simulink model "working_kalman"  (R2025b)
settings: Solver=FixedStepDiscrete  StartTime=0.0  StopTime=+inf  FixedStep=simulink_Ts  RelTol=1e-3  EnableMultiTasking=on
InitFcn:
  | InitSensorFusion
values from neighbouring files (symbols this model uses):
  acc_calib_matrix = [0.9990,0.0039,0.0028;4.2507e-04,0.9990,-0.0085;0.0015,0.0090,0.9997]    [InitSensorFusion.m]
  avg_order = 2    [InitSensorFusion.m]
  calibration_time = 10    [InitSensorFusion.m]
  d = 0.15*sqrt(2)/2    [InitSensorFusion.m]
  friction_offset = 0.0001    [InitSensorFusion.m]
  friction_slope = 20e-6    (= 2e-05)    [InitSensorFusion.m]
  g = 9.81    [InitSensorFusion.m]
  ground_true_g = 9.81275    [InitSensorFusion.m]
  Ic0 = Is0 + Iw0 - Iwg    [InitSensorFusion.m]
  ICM42_gyr_offset = [-0.1319, -0.6878, 0.1737]    [InitSensorFusion.m]
  ICM42_params = SUPER_PARAMS    [InitSensorFusion.m]
  init_acc_bias = [-0.0076;0.0233;0.0477]    [InitSensorFusion.m]
  init_P = P_initial    [InitSensorFusion.m]
  init_rot_quat = [0 0 0 1]'    [InitSensorFusion.m]
  Iwg = 315e-6    (= 0.000315)    [InitSensorFusion.m]
  kalman_Ts = 0.01    [InitSensorFusion.m]
  KV = 330    [InitSensorFusion.m]
  mc = mw + ms    (= 0.75)    [InitSensorFusion.m]
  sensor_Ts = 0.01    [InitSensorFusion.m]
  simulink_Ts = 0.01    [InitSensorFusion.m]
  stateInit = StateEnum.Initialization    [InitSensorFusion.m]
undefined symbols (not defined in the file or in its folder): acc_init_bias, init_time, StateEnum
libraries: mbedblockslib x25, simulink x12, nucleoutilitieslib x10, stmnucleof7lib x7, canmsglib x6, simulink_extras x2, visionstatistics x2
(part 2 of 2)

== system working_kalman/Sensor Calibration and Averaging/Subsystem2 ==
  g_vector : Inport
  Enable : EnablePort
  2-D Mean3 : visionstatistics/2-D Mean  run=on  reset_popup=Rising edge  directionMode=Each row  dimension=1  treatSBRowAsCol=on  outputLastDataTypeStr=Inherit: Same as accumulator  accumMode=Binary point scaling  accumWordLength=32  accumFracLength=0  accumLastDataTypeStr=fixdt([],32,0)  roiEnable=off  roiType=Rectangles  roiPortion=Entire ROI  roiOutput=Individual statistics for each ROI  roiFlag=off  roundingMode=Floor  overflowMode=off  accumDataTypeStr=fixdt([],32,0)  outputDataTypeStr=Inherit: Same as accumulator  outputMin=[]  outputMax=[]
  Cast To Boolean : DataTypeConversion  OutDataTypeStr=boolean  SaturateOnIntegerOverflow=off  RndMeth=Floor
  MATLAB Function1 : MATLAB Function  TreatAsAtomicUnit=on
  Sum : Sum  Inputs=|-+
  Sum of Elements : Sum  Inputs=+
  ground_true_g_vector : Constant  Value=[0; 0; -ground_true_g]  SampleTime=simulink_Ts
  g_mean : Outport
  acc_bias : Outport  Port=2
  wires:
  2-D Mean3/1 -> g_mean/1
  g_vector/1 -> MATLAB Function1/1(g_vector), Sum of Elements/1, Sum/2
  MATLAB Function1/1(g_scalar) -> 2-D Mean3/1
  Sum of Elements/1 -> Cast To Boolean/1
  Cast To Boolean/1 -> 2-D Mean3/2
  ground_true_g_vector/1 -> Sum/1
  Sum/1 -> acc_bias/1

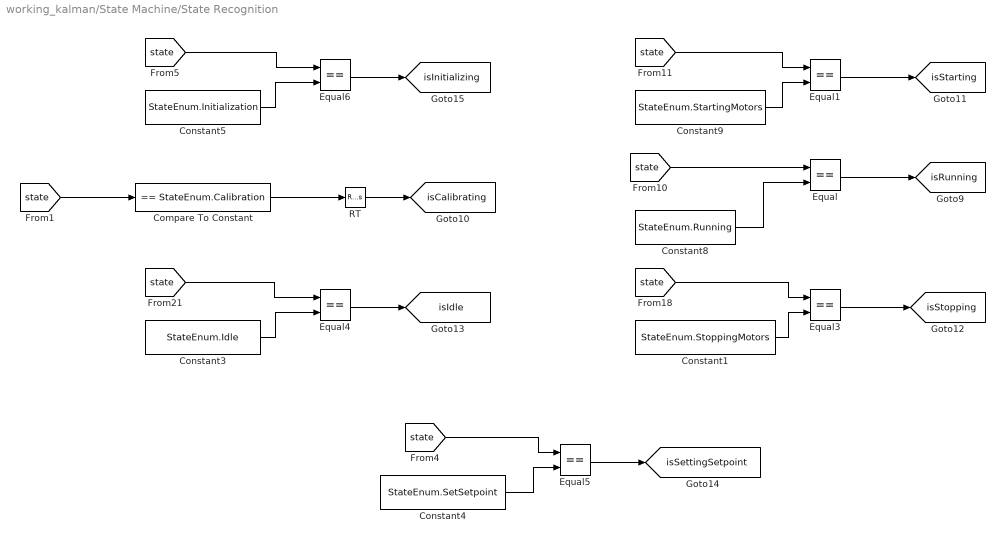
== system working_kalman/State Machine/State Recognition ==
  Compare To Constant : simulink/Logic and Bit Operations/Compare To Constant  relop===  const=StateEnum.Calibration  OutDataTypeStr=boolean
  Constant1 : Constant  Value=StateEnum.StoppingMotors  SampleTime=simulink_Ts
  Constant3 : Constant  Value=StateEnum.Idle  SampleTime=simulink_Ts
  Constant4 : Constant  Value=StateEnum.SetSetpoint  SampleTime=simulink_Ts
  Constant5 : Constant  Value=StateEnum.Initialization  SampleTime=simulink_Ts
  Constant8 : Constant  Value=StateEnum.Running  SampleTime=simulink_Ts
  Constant9 : Constant  Value=StateEnum.StartingMotors  SampleTime=simulink_Ts
  Equal{,1,3..6} (6 alike) : RelationalOperator  Operator===  OutDataTypeStr=boolean  RndMeth=Simplest  InputSameDT=off
  RT : RateTransition  OutPortSampleTime=sensor_Ts
  tag scope: isCalibrating=global, isIdle=global, isInitializing=global, isRunning=global, isSettingSetpoint=global, isStarting=global, isStopping=global
  wires:
  [state] -> Equal4/1
  Equal6/1 -> [isInitializing]
  [state] -> Equal1/1
  Constant9/1 -> Equal1/2
  Constant4/1 -> Equal5/2
  Constant8/1 -> Equal/2
  [state] -> Equal/1
  Equal4/1 -> [isIdle]
  Constant3/1 -> Equal4/2
  Constant5/1 -> Equal6/2
  Equal1/1 -> [isStarting]
  Equal/1 -> [isRunning]
  Constant1/1 -> Equal3/2
  [state] -> Equal3/1
  Equal5/1 -> [isSettingSetpoint]
  Equal3/1 -> [isStopping]
  [state] -> Equal6/1
  [state] -> Equal5/1
  [state] -> Compare To Constant/1
  Compare To Constant/1 -> RT/1
  RT/1 -> [isCalibrating]

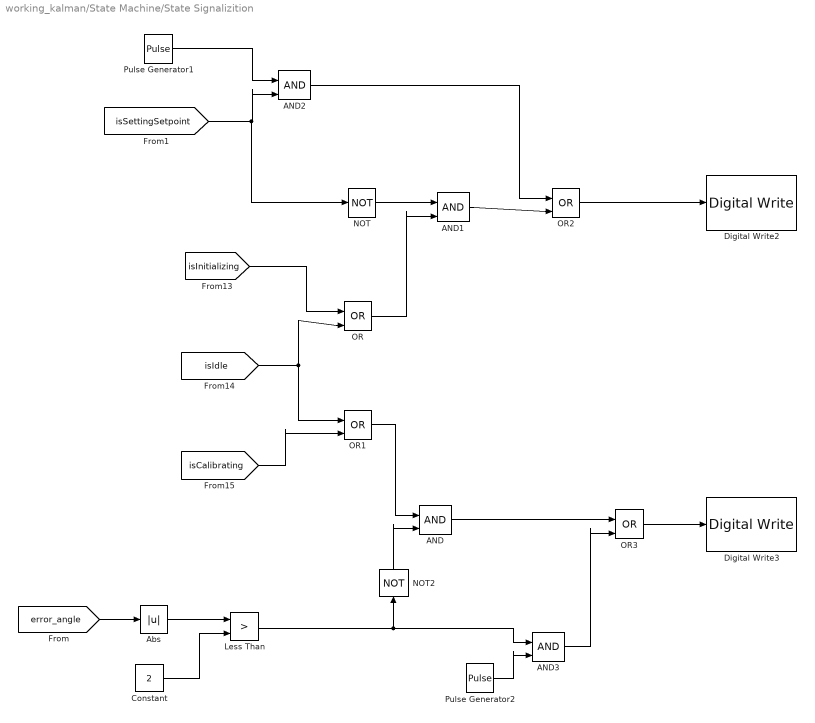
== system working_kalman/State Machine/State Signalizition ==
  AND{,1..3} (4 alike) : Logic  IconShape=distinctive  AllPortsSameDT=off  OutDataTypeStr=boolean
  Abs : Abs  SaturateOnIntegerOverflow=off
  Constant : Constant  Value=2
  Digital Write2 : mbedblockslib/Digital Write  Pin=LED3  Direction=output
      settings: LibrarySourceBlock=stmnucleorootlib/Common/Digital Write
  Digital Write3 : mbedblockslib/Digital Write  Pin=LED2  Direction=output
      settings: LibrarySourceBlock=stmnucleorootlib/Common/Digital Write
  Less Than : RelationalOperator  Operator=>  OutDataTypeStr=boolean  RndMeth=Simplest  InputSameDT=off
  NOT : Logic  Operator=NOT  IconShape=distinctive  AllPortsSameDT=off  OutDataTypeStr=boolean
  NOT2 : Logic  Operator=NOT  IconShape=distinctive  AllPortsSameDT=off  OutDataTypeStr=boolean
  OR{,1..3} (4 alike) : Logic  Operator=OR  IconShape=distinctive  AllPortsSameDT=off  OutDataTypeStr=boolean
  Pulse Generator1 : DiscretePulseGenerator  PulseType=Time based  Period=0.1  PulseWidth=50
  Pulse Generator2 : DiscretePulseGenerator  PulseType=Time based  Period=0.1  PulseWidth=50
  wires:
  [isInitializing] -> OR/1
  [isCalibrating] -> OR1/2
  [isIdle] -> OR1/1, OR/2
  OR1/1 -> AND/1
  OR/1 -> AND1/2
  Abs/1 -> Less Than/1
  Constant/1 -> Less Than/2
  Pulse Generator1/1 -> AND2/1
  [isSettingSetpoint] -> NOT/1, AND2/2
  NOT/1 -> AND1/1
  AND1/1 -> OR2/2
  AND2/1 -> OR2/1
  OR2/1 -> Digital Write2/1
  [error_angle] -> Abs/1
  Less Than/1 -> AND3/1, NOT2/1
  Pulse Generator2/1 -> AND3/2
  AND/1 -> OR3/1
  AND3/1 -> OR3/2
  OR3/1 -> Digital Write3/1
  NOT2/1 -> AND/2

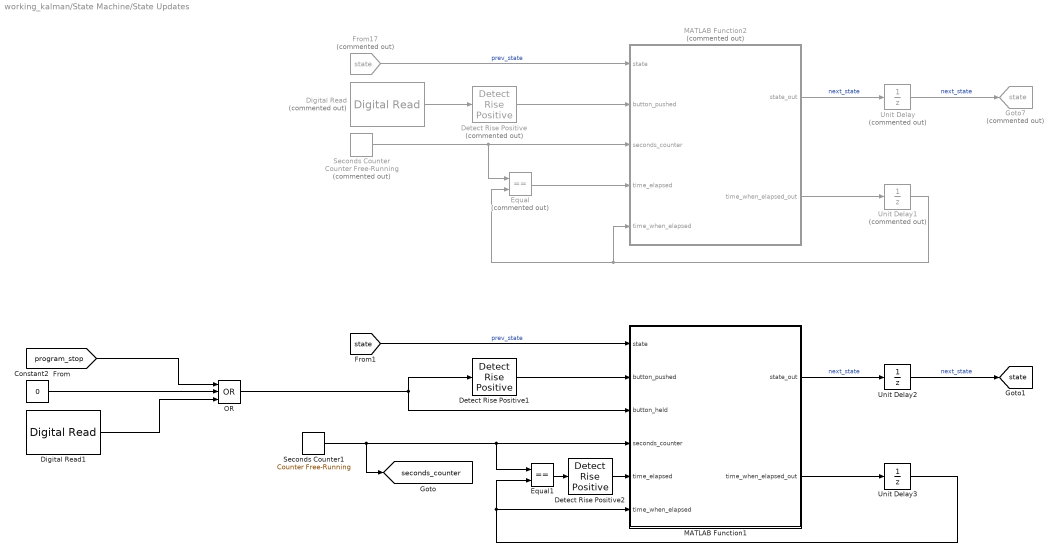
== system working_kalman/State Machine/State Updates ==
  Constant2 : Constant  Value=0
  Detect Rise Positive : simulink/Logic and Bit Operations/Detect Rise Positive  Commented=on  vinit=0  OutDataTypeStr=boolean
  Detect Rise Positive1 : simulink/Logic and Bit Operations/Detect Rise Positive  vinit=0  OutDataTypeStr=boolean
  Detect Rise Positive2 : simulink/Logic and Bit Operations/Detect Rise Positive  vinit=0  OutDataTypeStr=boolean
  Digital Read : mbedblockslib/Digital Read  Commented=on  Pin=D0  Direction=input  SampleTime=0.1
      settings: LibrarySourceBlock=stmnucleorootlib/Common/Digital Read
  Digital Read1 : mbedblockslib/Digital Read  Pin=PC_13  Direction=input  SampleTime=simulink_Ts
      settings: LibrarySourceBlock=stmnucleorootlib/Common/Digital Read
  Equal : RelationalOperator  Commented=on  Operator===  OutDataTypeStr=boolean  RndMeth=Simplest  InputSameDT=off
  Equal1 : RelationalOperator  Operator===  OutDataTypeStr=boolean  RndMeth=Simplest  InputSameDT=off
  From17 : From  Commented=on  GotoTag=state  TagVisibility=global
  Goto7 : Goto  Commented=on  GotoTag=state  TagVisibility=global
  MATLAB Function1 : MATLAB Function  TreatAsAtomicUnit=on  SystemSampleTime=simulink_Ts
  MATLAB Function2 : MATLAB Function  Commented=on  TreatAsAtomicUnit=on
  OR : Logic  Operator=OR  Inputs=3  IconShape=distinctive  AllPortsSameDT=off  OutDataTypeStr=boolean
  Seconds Counter : simulink/Sources/Counter Free-Running  Commented=on  NumBits=16  tsamp=1
  Seconds Counter1 : simulink/Sources/Counter Free-Running  NumBits=16  tsamp=1
  Unit Delay : UnitDelay  Commented=on  InitialCondition=stateInit  SampleTime=-1  HasFrameUpgradeWarning=on
  Unit Delay1 : UnitDelay  Commented=on  InitialCondition=init_time  SampleTime=-1  HasFrameUpgradeWarning=on
  Unit Delay2 : UnitDelay  InitialCondition=stateInit  SampleTime=simulink_Ts  HasFrameUpgradeWarning=on
  Unit Delay3 : UnitDelay  InitialCondition=init_time  SampleTime=simulink_Ts  HasFrameUpgradeWarning=on
  tag scope: seconds_counter=global, state=global
  wires:
  Unit Delay/1 -> Goto7/1  "next_state"
  Digital Read/1 -> Detect Rise Positive/1
  From17/1 -> MATLAB Function2/1(state)  "prev_state"
  Detect Rise Positive/1 -> MATLAB Function2/2(button_pushed)
  Seconds Counter/1 -> Equal/1, MATLAB Function2/3(seconds_counter)
  Equal/1 -> MATLAB Function2/4(time_elapsed)
  MATLAB Function2/2(time_when_elapsed_out) -> Unit Delay1/1
  Unit Delay1/1 -> MATLAB Function2/5(time_when_elapsed), Equal/2
  MATLAB Function2/1(state_out) -> Unit Delay/1  "next_state"
  Equal1/1 -> Detect Rise Positive2/1
  Detect Rise Positive1/1 -> MATLAB Function1/2(button_pushed)
  [state] -> MATLAB Function1/1(state)  "prev_state"
  Unit Delay2/1 -> [state]  "next_state"
  MATLAB Function1/1(state_out) -> Unit Delay2/1  "next_state"
  Seconds Counter1/1 -> Equal1/1, MATLAB Function1/4(seconds_counter), [seconds_counter]
  MATLAB Function1/2(time_when_elapsed_out) -> Unit Delay3/1
  Unit Delay3/1 -> Equal1/2, MATLAB Function1/6(time_when_elapsed)
  Constant2/1 -> OR/2
  [program_stop] -> OR/1
  Digital Read1/1 -> OR/3
  OR/1 -> Detect Rise Positive1/1, MATLAB Function1/3(button_held)
  Detect Rise Positive2/1 -> MATLAB Function1/5(time_elapsed)

== system working_kalman/CAN communication with B-G431-ESC1/Receive CAN Messages/Subsystem1 ==
  In1 : Inport
  Enable : EnablePort
  Byte Unpack : nucleoutilitieslib/Byte Unpack  dimensions={[2]}  datatypes={'single'}  byteAlign=1  blockPlatform=nucleo
  Out1 : Outport
  wires:
  Byte Unpack/1 -> Out1/1
  In1/1 -> Byte Unpack/1

== system working_kalman/CAN communication with B-G431-ESC1/Receive CAN Messages/Subsystem2 ==
  In1 : Inport
  Enable : EnablePort
  Byte Unpack : nucleoutilitieslib/Byte Unpack  dimensions={[2]}  datatypes={'single'}  byteAlign=1  blockPlatform=nucleo
  Out1 : Outport
  wires:
  Byte Unpack/1 -> Out1/1
  In1/1 -> Byte Unpack/1

== system working_kalman/CAN communication with B-G431-ESC1/Send CAN Messages/CAN_send ==
  data : Inport
  ID : Inport  Port=2
  Trigger : TriggerPort  VariantControl=(inherit)  PortDimensions=1
  CAN Pack : canmsglib/CAN Pack  MsgList=(none)  MsgName=LED_set  MsgIDType=Standard (11-bit identifier)  MsgIdentifier=hex2dec('7F3')  CANIDInput=on  MsgLength=8  Remote=off  ApplyMinMax=off  BusOutput=on  SignalInfo={}
      settings: LibrarySourceBlock=nucleoutilitieslib/CAN Pack  DataFormat=raw data
  CAN Transmit : stmnucleof7lib/CAN Transmit  CANModule=1  IdentifierType=Standard (11-bit identifier)  MsgId=hex2dec('7F3')  MsgLen=8  OutputStatus=on  RemoteFrame=off
      settings: DataFormat=CAN Message
  wires:
  CAN Pack/1 -> CAN Transmit/1
  data/1 -> CAN Pack/1
  ID/1 -> CAN Pack/2

== system working_kalman/CAN communication with B-G431-ESC1/Send CAN Messages/CAN_send1 ==
  data : Inport
  ID : Inport  Port=2
  Trigger : TriggerPort  VariantControl=(inherit)  PortDimensions=1
  CAN Pack : canmsglib/CAN Pack  MsgList=(none)  MsgName=LED_set  MsgIDType=Standard (11-bit identifier)  MsgIdentifier=hex2dec('7F3')  CANIDInput=on  MsgLength=8  Remote=off  ApplyMinMax=off  BusOutput=on  SignalInfo={}
      settings: LibrarySourceBlock=nucleoutilitieslib/CAN Pack  DataFormat=raw data
  CAN Transmit : stmnucleof7lib/CAN Transmit  CANModule=1  IdentifierType=Standard (11-bit identifier)  MsgId=hex2dec('7F3')  MsgLen=8  OutputStatus=on  RemoteFrame=off
      settings: DataFormat=CAN Message
  wires:
  CAN Pack/1 -> CAN Transmit/1
  data/1 -> CAN Pack/1
  ID/1 -> CAN Pack/2

== system working_kalman/CAN communication with B-G431-ESC1/Send CAN Messages/CAN_send2 ==
  data : Inport
  ID : Inport  Port=2
  Trigger : TriggerPort  VariantControl=(inherit)  PortDimensions=1
  CAN Pack : canmsglib/CAN Pack  MsgList=(none)  MsgName=LED_set  MsgIDType=Standard (11-bit identifier)  MsgIdentifier=hex2dec('7F3')  CANIDInput=on  MsgLength=8  Remote=off  ApplyMinMax=off  BusOutput=on  SignalInfo={}
      settings: LibrarySourceBlock=nucleoutilitieslib/CAN Pack  DataFormat=raw data
  CAN Transmit : stmnucleof7lib/CAN Transmit  CANModule=1  IdentifierType=Standard (11-bit identifier)  MsgId=hex2dec('7F3')  MsgLen=8  OutputStatus=on  RemoteFrame=off
      settings: DataFormat=CAN Message
  wires:
  CAN Pack/1 -> CAN Transmit/1
  data/1 -> CAN Pack/1
  ID/1 -> CAN Pack/2

== system working_kalman/CAN communication with B-G431-ESC1/Send CAN Messages/CAN_send3 ==
  data : Inport
  ID : Inport  Port=2
  Trigger : TriggerPort  VariantControl=(inherit)  PortDimensions=1
  CAN Pack : canmsglib/CAN Pack  MsgList=(none)  MsgName=LED_set  MsgIDType=Standard (11-bit identifier)  MsgIdentifier=hex2dec('7F3')  CANIDInput=on  MsgLength=8  Remote=off  ApplyMinMax=off  BusOutput=on  SignalInfo={}
      settings: LibrarySourceBlock=nucleoutilitieslib/CAN Pack  DataFormat=raw data
  CAN Transmit : stmnucleof7lib/CAN Transmit  CANModule=1  IdentifierType=Standard (11-bit identifier)  MsgId=hex2dec('7F3')  MsgLen=8  OutputStatus=on  RemoteFrame=off
      settings: DataFormat=CAN Message
  wires:
  CAN Pack/1 -> CAN Transmit/1
  data/1 -> CAN Pack/1
  ID/1 -> CAN Pack/2

== system working_kalman/CAN communication with B-G431-ESC1/Send CAN Messages/CAN_send4 ==
  data : Inport
  ID : Inport  Port=2
  Trigger : TriggerPort  VariantControl=(inherit)  PortDimensions=1
  CAN Pack : canmsglib/CAN Pack  MsgList=(none)  MsgName=LED_set  MsgIDType=Standard (11-bit identifier)  MsgIdentifier=hex2dec('7F3')  CANIDInput=on  MsgLength=8  Remote=off  ApplyMinMax=off  BusOutput=on  SignalInfo={}
      settings: LibrarySourceBlock=nucleoutilitieslib/CAN Pack  DataFormat=raw data
  CAN Transmit : stmnucleof7lib/CAN Transmit  CANModule=1  IdentifierType=Standard (11-bit identifier)  MsgId=hex2dec('7F3')  MsgLen=8  OutputStatus=on  RemoteFrame=off
      settings: DataFormat=CAN Message
  wires:
  CAN Pack/1 -> CAN Transmit/1
  data/1 -> CAN Pack/1
  ID/1 -> CAN Pack/2

== system working_kalman/CAN communication with B-G431-ESC1/Send CAN Messages/CAN_send5 ==
  data : Inport
  ID : Inport  Port=2
  Trigger : TriggerPort  VariantControl=(inherit)  PortDimensions=1
  CAN Pack : canmsglib/CAN Pack  MsgList=(none)  MsgName=LED_set  MsgIDType=Standard (11-bit identifier)  MsgIdentifier=hex2dec('7F3')  CANIDInput=on  MsgLength=8  Remote=off  ApplyMinMax=off  BusOutput=on  SignalInfo={}
      settings: LibrarySourceBlock=nucleoutilitieslib/CAN Pack  DataFormat=raw data
  CAN Transmit : stmnucleof7lib/CAN Transmit  CANModule=1  IdentifierType=Standard (11-bit identifier)  MsgId=hex2dec('7F3')  MsgLen=8  OutputStatus=on  RemoteFrame=off
      settings: DataFormat=CAN Message
  wires:
  CAN Pack/1 -> CAN Transmit/1
  data/1 -> CAN Pack/1
  ID/1 -> CAN Pack/2

== system working_kalman/CAN communication with B-G431-ESC1/Send CAN Messages/Set_LED ==
  Cast To Double : DataTypeConversion  OutDataTypeStr=uint8  SaturateOnIntegerOverflow=off  RndMeth=Floor
  Constant : Constant  Value=zeros(1,7)
  Constant5 : Constant  Value=hex2dec('7F3')
  Pulse Generator1 : DiscretePulseGenerator  PulseType=Time based  Period=1  PulseWidth=50
  Vector Concatenate : Concatenate
  data : Outport
  ID : Outport  Port=2
  wires:
  Constant5/1 -> ID/1
  Pulse Generator1/1 -> Vector Concatenate/1
  Vector Concatenate/1 -> Cast To Double/1
  Constant/1 -> Vector Concatenate/2
  Cast To Double/1 -> data/1

== system working_kalman/CAN communication with B-G431-ESC1/Send CAN Messages/Set_speed ==
  Byte Pack1 : nucleoutilitieslib/Byte Pack  datatypes={'uint16'}  byteAlign=1  blockPlatform=nucleo
  Byte Pack2 : nucleoutilitieslib/Byte Pack  datatypes={'single'}  byteAlign=1  blockPlatform=nucleo
  Constant1 : Constant  Value=[0,0]  OutDataTypeStr=uint8  SampleTime=-1
  Constant5 : Constant  Value=hex2dec('023')
  Vector Concatenate3 : Concatenate  NumInputs=3
  time_ramp [ms] : Constant  Value=0  OutDataTypeStr=uint16
  data : Outport
  ID : Outport  Port=2
  wires:
  Vector Concatenate3/1 -> data/1
  Constant5/1 -> ID/1
  Byte Pack2/1 -> Vector Concatenate3/1
  Byte Pack1/1 -> Vector Concatenate3/2
  Constant1/1 -> Vector Concatenate3/3
  time_ramp [ms]/1 -> Byte Pack1/1
  [ramp_speed] -> Byte Pack2/1

== system working_kalman/CAN communication with B-G431-ESC1/Send CAN Messages/Set_speed1 ==
  In1 : Inport
  Byte Pack1 : nucleoutilitieslib/Byte Pack  datatypes={'uint16'}  byteAlign=1  blockPlatform=nucleo
  Byte Pack2 : nucleoutilitieslib/Byte Pack  datatypes={'single'}  byteAlign=1  blockPlatform=nucleo
  Constant1 : Constant  Value=[0,0]  OutDataTypeStr=uint8  SampleTime=-1
  Constant5 : Constant  Value=hex2dec('023')
  Sum : Sum  Inputs=++|
  Vector Concatenate3 : Concatenate  NumInputs=3
  final_speed [rpm] : Constant  Value=1200  OutDataTypeStr=single
  time_ramp [ms] : Constant  Value=500  OutDataTypeStr=uint16
  data : Outport
  ID : Outport  Port=2
  wires:
  time_ramp [ms]/1 -> Byte Pack1/1
  Constant1/1 -> Vector Concatenate3/3
  Byte Pack1/1 -> Vector Concatenate3/2
  Byte Pack2/1 -> Vector Concatenate3/1
  Constant5/1 -> ID/1
  Vector Concatenate3/1 -> data/1
  final_speed [rpm]/1 -> Sum/2
  Sum/1 -> Byte Pack2/1
  In1/1 -> Sum/1  "angle_dep_spd"

== system working_kalman/CAN communication with B-G431-ESC1/Send CAN Messages/Set_torque ==
  Byte Pack1 : nucleoutilitieslib/Byte Pack  datatypes={'uint16'}  byteAlign=1  blockPlatform=nucleo
  Byte Pack2 : nucleoutilitieslib/Byte Pack  datatypes={'single'}  byteAlign=1  blockPlatform=nucleo
  Cast : DataTypeConversion  OutDataTypeStr=single  SaturateOnIntegerOverflow=off  RndMeth=Floor
  Constant1 : Constant  Value=[0,0]  OutDataTypeStr=uint8  SampleTime=-1
  Constant5 : Constant  Value=hex2dec('043')
  Vector Concatenate3 : Concatenate  NumInputs=3
  time_ramp [ms] : Constant  Value=0  OutDataTypeStr=uint16  SampleTime=-1
  data : Outport
  ID : Outport  Port=2
  wires:
  time_ramp [ms]/1 -> Byte Pack1/1
  Constant1/1 -> Vector Concatenate3/3
  Byte Pack1/1 -> Vector Concatenate3/2
  Byte Pack2/1 -> Vector Concatenate3/1
  Constant5/1 -> ID/1
  Vector Concatenate3/1 -> data/1
  [ramp_torque] -> Cast/1  "reference_torque [A]"
  Cast/1 -> Byte Pack2/1

== system working_kalman/CAN communication with B-G431-ESC1/Send CAN Messages/Start_Motor ==
  Constant3 : Constant  Value=[1,0,0,0,0,0,0,0]  OutDataTypeStr=uint8  SampleTime=-1
  Constant4 : Constant  Value=hex2dec('033')
  data : Outport
  ID : Outport  Port=2
  wires:
  Constant3/1 -> data/1
  Constant4/1 -> ID/1

== system working_kalman/CAN communication with B-G431-ESC1/Send CAN Messages/Stop_Motor ==
  Byte Pack1 : nucleoutilitieslib/Byte Pack  datatypes={'uint16'}  byteAlign=1  blockPlatform=nucleo
  Byte Pack2 : nucleoutilitieslib/Byte Pack  datatypes={'single'}  byteAlign=1  blockPlatform=nucleo
  Constant1 : Constant  Value=[0,0]  OutDataTypeStr=uint8  SampleTime=-1
  Constant3 : Constant  Value=[0,0,0,0,0,0,0,0]  OutDataTypeStr=uint8  SampleTime=-1
  Constant4 : Constant  Value=hex2dec('033')
  Constant5 : Constant  Value=hex2dec('023')
  Vector Concatenate3 : Concatenate  NumInputs=3
  final_speed [rpm] : Constant  Value=-1200  OutDataTypeStr=single
  time_ramp [ms] : Constant  OutDataTypeStr=uint16
  data : Outport
  ID : Outport  Port=2
  wires:
  Byte Pack2/1 -> Vector Concatenate3/1
  final_speed [rpm]/1 -> Byte Pack2/1
  time_ramp [ms]/1 -> Byte Pack1/1
  Byte Pack1/1 -> Vector Concatenate3/2
  Constant1/1 -> Vector Concatenate3/3
  Constant4/1 -> ID/1
  Constant3/1 -> data/1

== system working_kalman/ICM20948/Read sensing data/Subsystem ==
  In1 : Inport
  Add Constant : Bias  Bias=36.53  SaturateOnIntegerOverflow=off
  Cast To Double : DataTypeConversion  OutDataTypeStr=double  SaturateOnIntegerOverflow=off  RndMeth=Floor
  Gain7 : Gain  Gain=1/340
  Out1 : Outport
  wires:
  Gain7/1 -> Add Constant/1  "Temp"
  Add Constant/1 -> Out1/1
  In1/1 -> Cast To Double/1
  Cast To Double/1 -> Gain7/1

== system working_kalman/ICM20948/Read sensing data/Subsystem1 ==
  In1 : Inport
  8g range : Gain  Gain=9.81275/4096
  Cast To Double : DataTypeConversion  OutDataTypeStr=double  SaturateOnIntegerOverflow=off  RndMeth=Floor
  Offset : Bias  SaturateOnIntegerOverflow=off
  Out1 : Outport
  wires:
  Cast To Double/1 -> 8g range/1
  Offset/1 -> Out1/1
  In1/1 -> Cast To Double/1
  8g range/1 -> Offset/1  "Acc_Z"

== system working_kalman/ICM20948/Read sensing data/Subsystem2 ==
  In1 : Inport
  8g range : Gain  Gain=9.81275/4096
  Cast To Double : DataTypeConversion  OutDataTypeStr=double  SaturateOnIntegerOverflow=off  RndMeth=Floor
  Offset : Bias  SaturateOnIntegerOverflow=off
  Out1 : Outport
  wires:
  8g range/1 -> Offset/1  "Acc_Z"
  In1/1 -> Cast To Double/1
  Offset/1 -> Out1/1
  Cast To Double/1 -> 8g range/1

== system working_kalman/ICM20948/Read sensing data/Subsystem3 ==
  In1 : Inport
  8g range : Gain  Gain=9.81275/4096
  Cast To Double : DataTypeConversion  OutDataTypeStr=double  SaturateOnIntegerOverflow=off  RndMeth=Floor
  Offset : Bias  SaturateOnIntegerOverflow=off
  Out1 : Outport
  wires:
  8g range/1 -> Offset/1  "Acc_Z"
  In1/1 -> Cast To Double/1
  Offset/1 -> Out1/1
  Cast To Double/1 -> 8g range/1

== system working_kalman/ICM20948/Read sensing data/Subsystem4 ==
  In1 : Inport
  +-500 °/s range : Gain  Gain=1/65.5
  Cast To Double : DataTypeConversion  OutDataTypeStr=double  SaturateOnIntegerOverflow=off  RndMeth=Floor
  Offset : Bias  SaturateOnIntegerOverflow=off
  Out1 : Outport
  wires:
  Offset/1 -> Out1/1
  +-500 °/s range/1 -> Offset/1  "Acc_Z"
  Cast To Double/1 -> +-500 °/s range/1
  In1/1 -> Cast To Double/1

== system working_kalman/ICM20948/Read sensing data/Subsystem5 ==
  In1 : Inport
  +-500 °/s range : Gain  Gain=1/65.5
  Cast To Double : DataTypeConversion  OutDataTypeStr=double  SaturateOnIntegerOverflow=off  RndMeth=Floor
  Offset : Bias  SaturateOnIntegerOverflow=off
  Out1 : Outport
  wires:
  Offset/1 -> Out1/1
  +-500 °/s range/1 -> Offset/1  "Acc_Z"
  Cast To Double/1 -> +-500 °/s range/1
  In1/1 -> Cast To Double/1

== system working_kalman/ICM20948/Read sensing data/Subsystem6 ==
  In1 : Inport
  +-500 °/s range : Gain  Gain=1/65.5
  Cast To Double : DataTypeConversion  OutDataTypeStr=double  SaturateOnIntegerOverflow=off  RndMeth=Floor
  Offset : Bias  SaturateOnIntegerOverflow=off
  Out1 : Outport
  wires:
  Offset/1 -> Out1/1
  +-500 °/s range/1 -> Offset/1  "Acc_Z"
  Cast To Double/1 -> +-500 °/s range/1
  In1/1 -> Cast To Double/1

== system working_kalman/ICM42688-P/Measurement/Subsystem ==
  In1 : Inport
  Add Constant : Bias  Bias=25  SaturateOnIntegerOverflow=off
  Cast To Double : DataTypeConversion  OutDataTypeStr=double  SaturateOnIntegerOverflow=off  RndMeth=Floor
  Gain7 : Gain  Gain=1/132.48
  Out1 : Outport
  wires:
  Gain7/1 -> Add Constant/1  "Temp"
  Add Constant/1 -> Out1/1
  In1/1 -> Cast To Double/1
  Cast To Double/1 -> Gain7/1

== system working_kalman/ICM42688-P/Measurement/Subsystem1 ==
  In1 : Inport
  8g range : Gain  Gain=9.81275*16/(2^16-1)
  Cast To Double : DataTypeConversion  OutDataTypeStr=double  SaturateOnIntegerOverflow=off  RndMeth=Floor
  Offset : Bias  SaturateOnIntegerOverflow=off
  Out1 : Outport
  wires:
  Cast To Double/1 -> 8g range/1
  Offset/1 -> Out1/1
  In1/1 -> Cast To Double/1
  8g range/1 -> Offset/1  "Acc_X"

== system working_kalman/ICM42688-P/Measurement/Subsystem2 ==
  In1 : Inport
  8g range : Gain  Gain=9.81275*16/(2^16-1)
  Cast To Double : DataTypeConversion  OutDataTypeStr=double  SaturateOnIntegerOverflow=off  RndMeth=Floor
  Offset : Bias  SaturateOnIntegerOverflow=off
  Out1 : Outport
  wires:
  8g range/1 -> Offset/1  "Acc_Y"
  In1/1 -> Cast To Double/1
  Offset/1 -> Out1/1
  Cast To Double/1 -> 8g range/1

== system working_kalman/ICM42688-P/Measurement/Subsystem3 ==
  In1 : Inport
  8g range : Gain  Gain=9.81275*16/(2^16-1)
  Cast To Double : DataTypeConversion  OutDataTypeStr=double  SaturateOnIntegerOverflow=off  RndMeth=Floor
  Offset : Bias  SaturateOnIntegerOverflow=off
  Out1 : Outport
  wires:
  8g range/1 -> Offset/1  "Acc_Z"
  In1/1 -> Cast To Double/1
  Offset/1 -> Out1/1
  Cast To Double/1 -> 8g range/1

== system working_kalman/ICM42688-P/Measurement/Subsystem4 ==
  In1 : Inport
  +-1000 °/s range : Gain  Gain=2000/(2^16-1)
  Cast To Double : DataTypeConversion  OutDataTypeStr=double  SaturateOnIntegerOverflow=off  RndMeth=Floor
  Offset : Bias  SaturateOnIntegerOverflow=off
  Out1 : Outport
  wires:
  Offset/1 -> Out1/1
  +-1000 °/s range/1 -> Offset/1  "Gyr_X"
  Cast To Double/1 -> +-1000 °/s range/1
  In1/1 -> Cast To Double/1

== system working_kalman/ICM42688-P/Measurement/Subsystem5 ==
  In1 : Inport
  +-1000 °/s range1 : Gain  Gain=2000/(2^16-1)
  Cast To Double : DataTypeConversion  OutDataTypeStr=double  SaturateOnIntegerOverflow=off  RndMeth=Floor
  Offset : Bias  SaturateOnIntegerOverflow=off
  Out1 : Outport
  wires:
  Offset/1 -> Out1/1
  +-1000 °/s range1/1 -> Offset/1  "Gyr_Y"
  Cast To Double/1 -> +-1000 °/s range1/1
  In1/1 -> Cast To Double/1

== system working_kalman/ICM42688-P/Measurement/Subsystem6 ==
  In1 : Inport
  +-1000 °/s range : Gain  Gain=2000/(2^16-1)
  Cast To Double : DataTypeConversion  OutDataTypeStr=double  SaturateOnIntegerOverflow=off  RndMeth=Floor
  Offset : Bias  SaturateOnIntegerOverflow=off
  Out1 : Outport
  wires:
  Offset/1 -> Out1/1
  +-1000 °/s range/1 -> Offset/1  "Gyr_Z"
  Cast To Double/1 -> +-1000 °/s range/1
  In1/1 -> Cast To Double/1

== system working_kalman/MPU6050/Read sensing data/Subsystem ==
  In1 : Inport
  Add Constant : Bias  Bias=36.53  SaturateOnIntegerOverflow=off
  Cast To Double : DataTypeConversion  OutDataTypeStr=double  SaturateOnIntegerOverflow=off  RndMeth=Floor
  Gain7 : Gain  Gain=1/340
  Out1 : Outport
  wires:
  Gain7/1 -> Add Constant/1  "Temp"
  Add Constant/1 -> Out1/1
  In1/1 -> Cast To Double/1
  Cast To Double/1 -> Gain7/1

== system working_kalman/MPU6050/Read sensing data/Subsystem1 ==
  In1 : Inport
  8g range : Gain  Gain=9.81275/4096
  Cast To Double : DataTypeConversion  OutDataTypeStr=double  SaturateOnIntegerOverflow=off  RndMeth=Floor
  Offset : Bias  SaturateOnIntegerOverflow=off
  Out1 : Outport
  wires:
  Cast To Double/1 -> 8g range/1
  Offset/1 -> Out1/1
  In1/1 -> Cast To Double/1
  8g range/1 -> Offset/1  "Acc_Z"

== system working_kalman/MPU6050/Read sensing data/Subsystem2 ==
  In1 : Inport
  8g range : Gain  Gain=9.81275/4096
  Cast To Double : DataTypeConversion  OutDataTypeStr=double  SaturateOnIntegerOverflow=off  RndMeth=Floor
  Offset : Bias  SaturateOnIntegerOverflow=off
  Out1 : Outport
  wires:
  8g range/1 -> Offset/1  "Acc_Z"
  In1/1 -> Cast To Double/1
  Offset/1 -> Out1/1
  Cast To Double/1 -> 8g range/1

== system working_kalman/MPU6050/Read sensing data/Subsystem3 ==
  In1 : Inport
  8g range : Gain  Gain=9.81275/4096
  Cast To Double : DataTypeConversion  OutDataTypeStr=double  SaturateOnIntegerOverflow=off  RndMeth=Floor
  Offset : Bias  SaturateOnIntegerOverflow=off
  Out1 : Outport
  wires:
  8g range/1 -> Offset/1  "Acc_Z"
  In1/1 -> Cast To Double/1
  Offset/1 -> Out1/1
  Cast To Double/1 -> 8g range/1

== system working_kalman/MPU6050/Read sensing data/Subsystem4 ==
  In1 : Inport
  +-500 °/s range : Gain  Gain=1/65.5
  Cast To Double : DataTypeConversion  OutDataTypeStr=double  SaturateOnIntegerOverflow=off  RndMeth=Floor
  Offset : Bias  SaturateOnIntegerOverflow=off
  Out1 : Outport
  wires:
  Offset/1 -> Out1/1
  +-500 °/s range/1 -> Offset/1  "Acc_Z"
  Cast To Double/1 -> +-500 °/s range/1
  In1/1 -> Cast To Double/1

== system working_kalman/MPU6050/Read sensing data/Subsystem5 ==
  In1 : Inport
  +-500 °/s range : Gain  Gain=1/65.5
  Cast To Double : DataTypeConversion  OutDataTypeStr=double  SaturateOnIntegerOverflow=off  RndMeth=Floor
  Offset : Bias  SaturateOnIntegerOverflow=off
  Out1 : Outport
  wires:
  Offset/1 -> Out1/1
  +-500 °/s range/1 -> Offset/1  "Acc_Z"
  Cast To Double/1 -> +-500 °/s range/1
  In1/1 -> Cast To Double/1

== system working_kalman/MPU6050/Read sensing data/Subsystem6 ==
  In1 : Inport
  +-500 °/s range : Gain  Gain=1/65.5
  Cast To Double : DataTypeConversion  OutDataTypeStr=double  SaturateOnIntegerOverflow=off  RndMeth=Floor
  Offset : Bias  SaturateOnIntegerOverflow=off
  Out1 : Outport
  wires:
  Offset/1 -> Out1/1
  +-500 °/s range/1 -> Offset/1  "Acc_Z"
  Cast To Double/1 -> +-500 °/s range/1
  In1/1 -> Cast To Double/1

== matlab function working_kalman/torque_stairs ==
  data: sampling_counter input; wheel_speed input; state input; step_done input; target_torque output; stop_start output; calibration_time parameter; init_time parameter; simulink_Ts parameter; t_in_slot output; step_done output
function [target_torque, stop_start, t_in_slot, step_done] = fcn(sampling_counter, wheel_speed, state, step_done, calibration_time, init_time, simulink_Ts)
%#codegen


seconds = double(sampling_counter) * simulink_Ts;

max_torque = -0.11;
torque_step = -0.005;
max_speed = 3500;

step_duration = 10;
rest_duration = 15;

num_steps      = round(max_torque / torque_step);

experiment_start = calibration_time + init_time;
t = seconds - experiment_start;  % time since experiment started
t_in_slot = 0;

% Default outputs
target_torque = 0;
stop_start    = 0;

if t < 0
    % Still in calibration / init phase
    return;
end

slot_duration = step_duration + rest_duration;  % max slot length
current_step  = floor(t / slot_duration);        % 0-indexed
t_in_slot     = t - double(current_step) * slot_duration;

if current_step >= num_steps
    stop_start    = 1;
    return;
end

target_torque = (double(current_step) + 1) * torque_step;

if (t_in_slot < simulink_Ts && step_done)
    step_done = 0;
end

if (t_in_slot < step_duration && abs(wheel_speed) < abs(max_speed) && ~step_done)
    % --- RUNNING phase ---
    % Send start signal at the very beginning of the slot
    if (state == StateEnum.Idle)
        stop_start = 1;   % start
    else
        stop_start = 0;
    end

elseif (t_in_slot >= step_duration || abs(wheel_speed) >= abs(max_speed))
    % --- STOP + REST phase ---
    % Send stop signal at the transition moment
    if (state == StateEnum.Running && t_in_slot > 1)
        stop_start = 1;  % stop
        step_done = 1;
    else
        stop_start = 0;
    end
    target_torque = 0;    % no torque during rest
end
end

== matlab function working_kalman/torque_inv_function ==
  data: desired_torque input; corrected_torque output; torque_inv_function parameter
function corrected_torque = fcn(desired_torque, torque_inv_function)
%#codegen

corrected_torque = polyval(torque_inv_function,desired_torque);

== matlab function working_kalman/Iq_peak_for_start ==
  data: desired_Iq input; Iq_for_start output; t_in_slot input; decay_slope input
function Iq_for_start = fcn(desired_Iq, t_in_slot, decay_slope)
%#codegen

pulse_amplitude = 0;

Iq_needed_for_start = 1*sign(desired_Iq);

if desired_Iq < 0
    pulse_amplitude = min((Iq_needed_for_start - desired_Iq),0);
elseif desired_Iq >= 0
    pulse_amplitude = max((Iq_needed_for_start - desired_Iq),0);
end

Iq_for_start = exp(-t_in_slot*decay_slope)*pulse_amplitude;

if(abs(Iq_for_start) < 0.01)
    Iq_for_start = 0;
end

== matlab function working_kalman/Iq_peak_for_start1 ==
  data: desired_Iq input; Iq_for_start output; t_in_slot input; decay_slope input
function Iq_for_start = fcn(desired_Iq, t_in_slot, decay_slope)
%#codegen

pulse_amplitude = 0;

Iq_needed_for_start = 1*sign(desired_Iq);

if desired_Iq < 0
    pulse_amplitude = min((Iq_needed_for_start - desired_Iq),0);
elseif desired_Iq >= 0
    pulse_amplitude = max((Iq_needed_for_start - desired_Iq),0);
end

Iq_for_start = exp(-t_in_slot*decay_slope)*pulse_amplitude;

if(abs(Iq_for_start) < 0.01)
    Iq_for_start = 0;
end

== matlab function working_kalman/torque_inv_function1 ==
  data: desired_torque input; corrected_torque output; torque_inv_function parameter
function corrected_torque = fcn(desired_torque, torque_inv_function)
%#codegen

corrected_torque = polyval(torque_inv_function,desired_torque);

== matlab function working_kalman/torque_stairs1 ==
  data: sampling_counter input; wheel_speed input; state input; step_done input; target_torque output; stop_start output; calibration_time parameter; init_time parameter; simulink_Ts parameter; t_in_slot output; step_done output
function [target_torque, stop_start, t_in_slot, step_done] = fcn(sampling_counter, wheel_speed, state, step_done, calibration_time, init_time, simulink_Ts)
%#codegen


seconds = double(sampling_counter) * simulink_Ts;

max_torque = 0.05;
torque_step = 0.002;
max_speed = 3500;

step_duration = 10;
rest_duration = 15;

num_steps      = round(max_torque / torque_step);

experiment_start = calibration_time + init_time;
t = seconds - experiment_start;  % time since experiment started
t_in_slot = 0;

% Default outputs
target_torque = 0;
stop_start    = 0;

if t < 0
    % Still in calibration / init phase
    return;
end

slot_duration = step_duration + rest_duration;  % max slot length
current_step  = floor(t / slot_duration);        % 0-indexed
t_in_slot     = t - double(current_step) * slot_duration;

if current_step >= num_steps
    stop_start    = 1;
    return;
end

target_torque = (double(current_step) + 1) * torque_step;

if (t_in_slot < simulink_Ts && step_done)
    step_done = 0;
end

if (t_in_slot < step_duration && abs(wheel_speed) < abs(max_speed) && ~step_done)
    % --- RUNNING phase ---
    % Send start signal at the very beginning of the slot
    if (state == StateEnum.Idle)
        stop_start = 1;   % start
    else
        stop_start = 0;
    end

elseif (t_in_slot >= step_duration || abs(wheel_speed) >= abs(max_speed))
    % --- STOP + REST phase ---
    % Send stop signal at the transition moment
    if (state == StateEnum.Running && t_in_slot > 1)
        stop_start = 1;  % stop
        step_done = 1;
    else
        stop_start = 0;
    end
    target_torque = 0;    % no torque during rest
end
end

== matlab function working_kalman/Iq_peak_for_start2 ==
  data: desired_Iq input; Iq_for_start output; t_in_slot input; decay_slope input
function Iq_for_start = fcn(desired_Iq, t_in_slot, decay_slope)
%#codegen

pulse_amplitude = 0;

Iq_needed_for_start = 1*sign(desired_Iq);

if desired_Iq < 0
    pulse_amplitude = min((Iq_needed_for_start - desired_Iq),0);
elseif desired_Iq >= 0
    pulse_amplitude = max((Iq_needed_for_start - desired_Iq),0);
end

Iq_for_start = exp(-t_in_slot*decay_slope)*pulse_amplitude;

if(abs(Iq_for_start) < 0.01)
    Iq_for_start = 0;
end

== matlab function working_kalman/torque_inv_function2 ==
  data: desired_torque input; corrected_torque output; torque_inv_function parameter
function corrected_torque = fcn(desired_torque, torque_inv_function)
%#codegen

corrected_torque = polyval(torque_inv_function,desired_torque);

== matlab function working_kalman/torque_stairs2 ==
  data: sampling_counter input; wheel_speed input; state input; step_done input; target_torque output; stop_start output; calibration_time parameter; init_time parameter; simulink_Ts parameter; t_in_slot output; step_done output
function [target_torque, stop_start, t_in_slot, step_done] = fcn(sampling_counter, wheel_speed, state, step_done, calibration_time, init_time, simulink_Ts)
%#codegen


seconds = double(sampling_counter) * simulink_Ts;

max_torque = 0.05;
torque_step = 0.002;
max_speed = 3500;

step_duration = 10;
rest_duration = 15;

num_steps      = round(max_torque / torque_step);

experiment_start = calibration_time + init_time;
t = seconds - experiment_start;  % time since experiment started
t_in_slot = 0;

% Default outputs
target_torque = 0;
stop_start    = 0;

if t < 0
    % Still in calibration / init phase
    return;
end

slot_duration = step_duration + rest_duration;  % max slot length
current_step  = floor(t / slot_duration);        % 0-indexed
t_in_slot     = t - double(current_step) * slot_duration;

if current_step >= num_steps
    stop_start    = 1;
    return;
end

target_torque = (double(current_step) + 1) * torque_step;

if (t_in_slot < simulink_Ts && step_done)
    step_done = 0;
end

if (t_in_slot < step_duration && abs(wheel_speed) < abs(max_speed) && ~step_done)
    % --- RUNNING phase ---
    % Send start signal at the very beginning of the slot
    if (state == StateEnum.Idle)
        stop_start = 1;   % start
    else
        stop_start = 0;
    end

elseif (t_in_slot >= step_duration || abs(wheel_speed) >= abs(max_speed))
    % --- STOP + REST phase ---
    % Send stop signal at the transition moment
    if (state == StateEnum.Running && t_in_slot > 1)
        stop_start = 1;  % stop
        step_done = 1;
    else
        stop_start = 0;
    end
    target_torque = 0;    % no torque during rest
end
end

== matlab function working_kalman/Torque Correction/torque_inv_function3 ==
  settings: updateMethod=DISCRETE  sampleTime=simulink_Ts
  data: desired_torque input; corrected_torque output; torque_inv_function parameter
function corrected_torque = fcn(desired_torque, torque_inv_function)
%#codegen

corrected_torque = polyval(torque_inv_function,desired_torque);

== matlab function working_kalman/Kalman Sensor Fusion for ICM42/Quat_to_YawPitchRoll ==
  settings: updateMethod=DISCRETE  sampleTime=kalman_Ts
  data: Q input; EA output
function EA = Quat2EulerAngles(Q)
%#codegen
% Vstup: Q = [q1, q2, q3, q4] kde q4 je skalár
% Výstup: EA = [Yaw, Pitch, Roll] v stupních

q1 = Q(1);
q2 = Q(2);
q3 = Q(3);
q4 = Q(4); % skalár

EA = [atan2d( 2*(q4*q3 + q1*q2),  1 - 2*(q2^2 + q3^2)); ...  % Yaw
      asind(  2*(q4*q2 - q3*q1));                          ... % Pitch
      atan2d( 2*(q4*q1 + q2*q3),  1 - 2*(q1^2 + q2^2))];     % Roll

if ~isreal(EA)
    EA = real(EA);
end

% Posun úhlu ROLL z -180 do 0
if EA(3) < 0
    EA(3) = EA(3) + 180;
else
    EA(3) = EA(3) - 180;
end


end

== matlab function working_kalman/Kalman Sensor Fusion for ICM42/Kalman Sensor Fusion for ICM42688-P ==
  settings: updateMethod=DISCRETE  sampleTime=kalman_Ts
  data: data input; rot_quat_out output; acc_bias_out output; IMU_Fs input; Param input; g input; P_out output; rot_quat input; acc_bias input; P input; trc_P output; std_acc output; K output; using_acc output
function [rot_quat_out, acc_bias_out, P_out, trc_P, std_acc, K, using_acc]  = Kalman_Sensor_Fusion_for_ICM42688_P(data, IMU_Fs, Param, g, rot_quat, acc_bias, P)
%#codegen

% This function implements  the sensor fusion algorithm proposed in
% "Quaternion-Based Extended Kalman Filter for Determining Orientation by Inertial and Magnetic Sensing"
% by Angelo M. Sabatini, IEEE TRANSACTIONS ON BIOMEDICAL ENGINEERING, VOL. 53, NO. 7, JULY 2006
% &
% Estimating Three-Dimensional Orientation of Human Body Parts by Inertial/Magnetic Sensing
% by Angelo Maria Sabatini, Sensors 2011, 11, 1489-1525; doi:10.3390/s110201489

%%% This code originally implemented by
% Marco Caruso (Politecnico di Torino), marco.caruso@studenti.polito.it
% Date: 21/11/2019

% The ORIGINAL code was modified by Milad Nazarahari
% (nazaraha@ualberta.ca), during Ph.D. studies under supervision of Dr. H. Rouhani
% (hrouhani@ualberta.ca), University of Alberta, December 2020 as a part of
% a comparative/benchmarking study.

% The MATLAB code performs the operations of the ORIGINAL code except for:
% reference acceleration/magnetic field (Earth's magnetic field)
% was obtained from sensor readout during motionless perioed at the begining of the experiment
% & implementing adaptive parameter tuning (hard-switch) & accelerometer and
% magnetometer bias were added as states

%  --------------- INPUT ---------------
%%%% "data" including
% acc            = 1x3 (m/s^2)
% gyr            = 1x3 (rad/s)
% Fs             = sampling frequency of the IMU (Hz)
% QS             = 1x2 (s) motionless period at the begining of the trial

%%%% Params
% (1,1) SIGMA_g        = gyrsocope noise for process noise covariance matrix static
% (1,2) SIGMA_g        = gyrsocope noise for process noise covariance matrix dynamic
% (1,3) epsilon_g      = threshold for switching between (1,1) & (1,2)
% (1,4) stdBiasAcc_in  = 1x1 (m/s^2) initial value for Accelerometer bias covariance matrix
% (1,5) stdAcc         = accelerometer noise for measurement noise covariance matrix static
% (1,6) stdAcc         = accelerometer noise for measurement noise covariance matrix dynamic
% (1,7) epsilon_a      = threshold for switching between (1,5) & (1,6)

% --------------- OUTPUT ---------------
% rot_quat             = Nx4 [qx qy qz qw], the scalar part is at the END of the quaternion


%-------------NEEDS TO BE INITIALIAZED-----------------

% rot_quat = zeros(len, 4);
% P = Param(1)*eye(7); % initial error covariance matrix
% g = norm(mean(accel(QS(1)*IMU_Fs:QS(2)*IMU_Fs, :))); % gravitational acceleration


accel = data(1:3);
gyro = deg2rad(data(4:6));
% len = size(accel,1);
dt = 1/IMU_Fs;

quaternion = [rot_quat' acc_bias']';

% PROCESS NOISE
SIGMA_a = dt*Param(4)^2*eye(3);



    % Updating Gyro noise adaptively (Q)
    if norm(gyro) <= Param(3)
        std_gyr = Param(1);
    else
        std_gyr = Param(2);
    end

    % std_gyr = Param(1) - norm(gyro)*Param(2);

    SIGMA_g = std_gyr^2*eye(3);
    
    %%%%%%%%%%%%%%%%%%%%%%%%%%%%% PREDICTION %%%%%%%%%%%%%%%%%%%%%%%%%%%%%%%%
    wx = gyro(1); wy = gyro(2); wz = gyro(3);
    omega = 0.5*[0    wz -wy wx
        -wz    0     wx wy
        wy -wx    0    wz
        -wx -wy -wz  0];%skew symmetric

    % omega = 0.5*[0    -wz wy wx
    %     wz    0     -wx wy
    %     -wy wx    0    wz
    %     -wx -wy -wz  0];%skew symmetric


    Phi = [expm(omega*dt) zeros(4,3);
           zeros(3,4)     eye(3)     ];
    
    % Project the state ahead
    quaternion_ = Phi*quaternion;
    
    CSI = [[0 -quaternion(3) quaternion(2);
        quaternion(3) 0 -quaternion(1);
        -quaternion(2) quaternion(1) 0]+quaternion(4)*eye(3);...
        -quaternion(1:3)'];
    
    Q = [(dt/2)^2*CSI*SIGMA_g*CSI' zeros(4,3);
        zeros(3,4) SIGMA_a      ];
    
    % Compute the a priori covariance matrix
    P_= Phi*P*Phi'+Q;
    
    %%%%%%%%%%%%%%%%%%%%%%%%%%%%% UPDATE STEP %%%%%%%%%%%%%%%%%%%%%%%%%%%%%%%%
    q1 = quaternion_(1); q2 = quaternion_(2); q3 = quaternion_(3); q4 = quaternion_(4);
    
    % Linearize the measurement equation: Jacobian
    F = [2*g*[q3 -q4 q1 -q2
        q4 q3 q2 q1
        -q1 -q2 q3 q4],eye(3)];
        
    
    % Adapt the measurement covariance matrix
    C = [q1^2-q2^2-q3^2+q4^2 2*(q1*q2+q3*q4) 2*(q1*q3-q2*q4)
        2*(q1*q2-q3*q4) -q1^2+q2^2-q3^2+q4^2 2*(q2*q3+q1*q4)
        2*(q1*q3+q2*q4) 2*(q2*q3-q1*q4) -q1^2-q2^2+q3^2+q4^2];
    
    criterion = norm(accel' - C*[0;0;g] - quaternion_(5:7));
    criterion = norm(accel) - g;
    criterion = norm(accel - C*[0;0;g] - quaternion_(5:7));

    % Accelerometer
    if (norm(accel) - g) < Param(7) % (Eq 70 in 2011 paper)  - quaternion_(5:7)
    % if (norm(accel) - g) < Param(7)
        std_acc = Param(5);
        using_acc = true;
    else
        std_acc = Param(6);
        using_acc = false;
    end
    % std_acc = Param(5) + criterion*Param(6)/g;
    
    % Measurement covariance
    R = std_acc^2*eye(3);
    
    % Compute the Kalman Gain
    K = P_* F' * (F * P_ * F' + R)^-1;
    
    % Compute the a posteriori state estimate
    z = accel; % measurement vector
    z_predict = C*[0; 0; g]; %+ quaternion_(5:end);
    quaternion = quaternion_ + K*(z - z_predict);
    
    % Normalize the quaternion
    quaternion(1:4) = quaternion(1:4)/norm(quaternion(1:4));
    
    % Compute the a posteriori covariance matrix
    P_out = P_ - K*F*P_;
    
    rot_quat_out = quaternion(1:4);
    acc_bias_out = quaternion(5:7);
    
    trc_P = trace(P_out);
    diff = norm(z - z_predict);
    
end

== matlab function working_kalman/Kalman Sensor Fusion for ICM42/Yaw Zeroing ==
  data: q input; q_out output
function q_out = fcn(q)
%#codegen

q_out = [0;0;0;1];

% Extrahuj Yaw
yaw = atan2(2*(q(4)*q(3) + q(1)*q(2)), ...
            1 - 2*(q(2)^2 + q(3)^2));

% Sestav kvaternion pro Yaw = -yaw (kompenzace)
q_yaw_inv = [cos(yaw/2); 0; 0; -sin(yaw/2)];

q = [q(4), q(1:3)']';

% Vynásob - odstraní Yaw složku
q_zeroed = quatmultiply(q_yaw_inv', q');

q_zeroed = [q_zeroed(2:4), q_zeroed(1)]';

q_out = q_zeroed / norm(q_zeroed);

== matlab function working_kalman/Sensor Calibration and Averaging/Subsystem2/MATLAB Function1 ==
  data: g_vector input; g_scalar output
function g_scalar = norm(g_vector)


g_scalar = norm(g_vector);

== matlab function working_kalman/Sensor Calibration and Averaging/MATLAB Function1 ==
  data: u input size=[1, 6]; avg output size=[6, 1]; avg_w input size=[avg_order,6]; avg_w output; avg_order parameter
function [avg, avg_w] = mov_avg(u, avg_w, avg_order)


% avg_order = 4;

avg_w = [u; avg_w(1:avg_order - 1,:)];

avg = mean(avg_w)';

== matlab function working_kalman/State Machine/State Updates/MATLAB Function2 ==
  data: state input Enum: StateEnum size=1; button_pushed input; seconds_counter input; state_out output Enum: StateEnum; time_elapsed input; time_when_elapsed input uint16; time_when_elapsed_out output uint16; calibration_time parameter

function [state_out, time_when_elapsed_out] = updateState(state, button_pushed, seconds_counter, time_elapsed, time_when_elapsed, calibration_time)
%#codegen
    
    state_out = state;
    time_when_elapsed_out = time_when_elapsed;

    switch(state)
        case StateEnum.Initialization
            if(time_elapsed)
                state_out = StateEnum.Calibration;
                time_when_elapsed_out = seconds_counter + calibration_time;
            end

        case StateEnum.Calibration
            if(time_elapsed)
                state_out = StateEnum.Idle;
            end

        case StateEnum.Idle
            if(button_pushed)
                state_out = StateEnum.StartingMotors;
            end

        case StateEnum.StartingMotors
            state_out = StateEnum.Running;
        
        case StateEnum.Running
            if(button_pushed)
                state_out = StateEnum.StoppingMotors;
            end

        case StateEnum.StoppingMotors
            state_out = StateEnum.Idle;
        
        case StateEnum.Error
    end
end

== matlab function working_kalman/State Machine/State Updates/MATLAB Function1 ==
  settings: updateMethod=DISCRETE  sampleTime=simulink_Ts
  data: state input Enum: StateEnum size=1; button_pushed input; button_held input; seconds_counter input; state_out output Enum: StateEnum; time_elapsed input; time_when_elapsed input uint16; time_when_elapsed_out output uint16; calibration_time parameter

function [state_out, time_when_elapsed_out] = updateState(state, button_pushed, button_held, seconds_counter, time_elapsed, time_when_elapsed, calibration_time)
%#codegen
    
    state_out = state;
    time_when_elapsed_out = time_when_elapsed;

    switch(state)
        case StateEnum.Initialization
            if(time_elapsed)
                state_out = StateEnum.Calibration;
                time_when_elapsed_out = seconds_counter + calibration_time;
            end

        case StateEnum.Calibration
            if(time_elapsed)
                state_out = StateEnum.Idle;
            end

        case StateEnum.Idle
            if(button_pushed)
                time_when_elapsed_out = seconds_counter + 1;
            end
            
            if(time_elapsed)
                if(~button_held)
                    state_out = StateEnum.StartingMotors;
                else
                    state_out = StateEnum.SetSetpoint;
                    time_when_elapsed_out = seconds_counter + 2;
                end
            end

        case StateEnum.StartingMotors
            state_out = StateEnum.Running;
        
        case StateEnum.Running
            if(button_pushed)
                state_out = StateEnum.StoppingMotors;
            end

        case StateEnum.StoppingMotors
            state_out = StateEnum.Idle;
        
        case StateEnum.SetSetpoint
             if(time_elapsed)
                state_out = StateEnum.Idle;
            end
    end
end

== matlab function working_kalman/speed_stairs_function ==
  data: seconds input; target_speed output; stop_start output; calibration_time parameter; init_time parameter
function [target_speed, stop_start] = fcn(seconds, calibration_time, init_time)
%#codegen

max_speed = 4000;
speed_step = 100;
step_duration = 10;

num_steps = max_speed / speed_step;         % 40 steps
total_time = num_steps * step_duration;     % 400 seconds

if seconds == (5 + calibration_time + init_time)
    stop_start = 1;
elseif seconds >= (total_time + calibration_time + init_time)
    stop_start = 1;
else
    stop_start = 0;
end

if seconds <= 0
    target_speed = 0;
elseif seconds >= (total_time + calibration_time + init_time)
    target_speed = 4000;
else
    step_index = ceil(seconds / step_duration);  % which step are we on
    step_index = min(step_index, num_steps);     % clamp to max
    target_speed = double(step_index) * speed_step;
end
